simulink model "DCMotorMEXNoControl"  (R2022b)
settings: Solver=VariableStepAuto  StartTime=0.0  StopTime=30  RelTol=1e-3
settings Model: Creator=Ananda Tjakra  LastModifiedBy=anand
settings SolverCC: AlgebraicLoopSolver=TrustRegion
settings DebuggingCC: UnconnectedInputMsg=warning  UnconnectedOutputMsg=warning  UnconnectedLineMsg=warning  SFMachineParentedDataDiag=warning
settings ModelReferenceCC: EnableRefExpFcnMdlSchedulingChecks=on

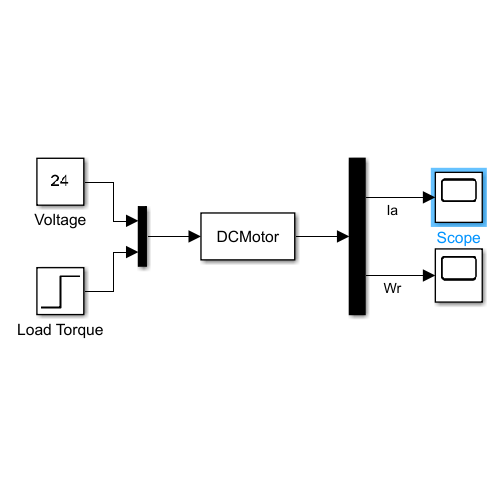
[thumbnail: Simulink's stored preview of the top-level diagram]
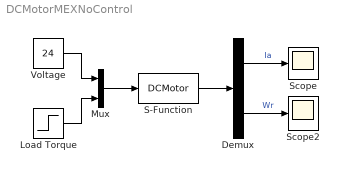
== system DCMotorMEXNoControl ==
  Demux : Demux  Outputs=2
  Load Torque : Step  Time=4  After=0  SampleTime=0
  Mux : Mux  Inputs=2
  S-Function : S-Function  FunctionName=DCMotor  SFunctionDeploymentMode=off  EnableBusSupport=off
  Scope : Scope
  Scope2 : Scope
  Voltage : Constant  Value=24
  wires:
  S-Function/1 -> Demux/1
  Mux/1 -> S-Function/1
  Voltage/1 -> Mux/1
  Load Torque/1 -> Mux/2
  Demux/1 -> Scope/1  "Ia"
  Demux/2 -> Scope2/1  "Wr"
